simulink model "actuator_control_with_torque_commands"  (R2015a)
settings: Solver=FixedStepDiscrete  StartTime=0.0  StopTime=inf  FixedStep=sample_time  RelTol=1e-3
undefined symbols (not defined in the file): A1_notch_f1, A2_notch_f1, B1_notch_f1, B2_notch_f1, fdesignblkfcn, gcbh, K_notch_f1, k_sea_low, lateral_motor_efficiency, max_sagittal_unloaded_torque, sample_time
libraries: slrtlib x4
settings Model: CovSFcnEnable=off  Creator=wmartin  LastModifiedBy=wmartin
settings SolverCC: EnableConcurrentExecution=on
settings DataIOCC: MaxDataPoints=1000000000  SaveFormat=StructureWithTime  SaveOutput=off  SaveTime=off
settings OptimizationCC: BlockReduction=off  OptimizeBlockIOStorage=off  BufferReuse=off  GlobalBufferReuse=off  ExpressionFolding=off  LocalBlockOutputs=off  SimCompilerOptimization=on
settings DebuggingCC: SolverPrmCheckMsg=warning
settings HardwareCC: ProdIntDivRoundTo=Zero  ProdEndianess=LittleEndian  ProdLongLongMode=on  ProdHWDeviceType=Generic->32-bit x86 compatible
settings ModelReferenceCC: UpdateModelReferenceTargets=AssumeUpToDate  ModelReferenceNumInstancesAllowed=Single  ModelReferenceMinAlgLoopOccurrences=on
settings RTWCC: SystemTargetFile=slrt.tlc  TemplateMakefile=slrt_default_tmf  Description=Simulink Real-Time  RTWVerbose=off  RTWCompilerOptimization=on
settings SimulinkRealTimeCC: GeneratePreprocessorConditionals=Disable all

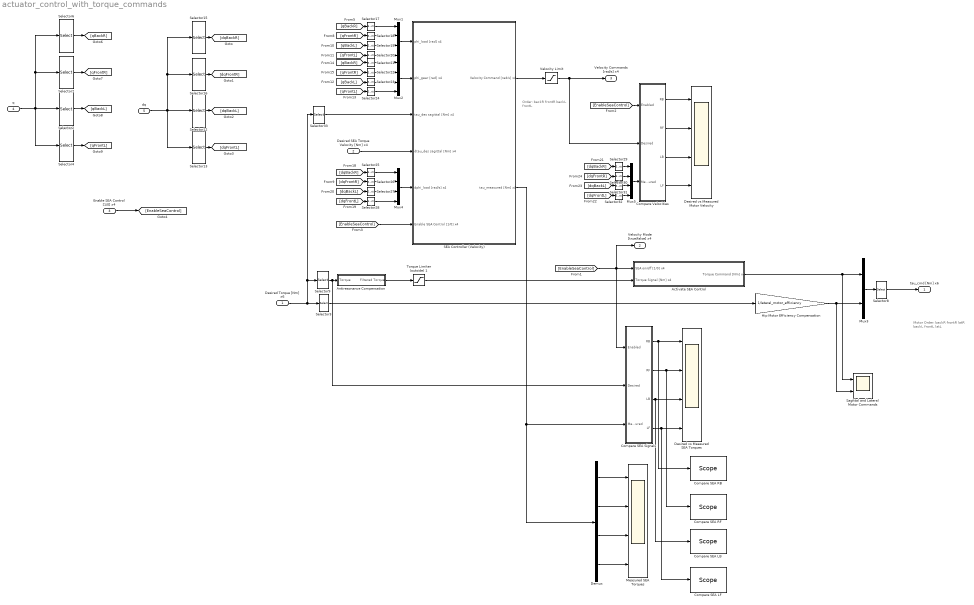
== system actuator_control_with_torque_commands ==
  note: Order:
      | backR
      | frontR
      | backL
      | frontL
  note: Motor Order:
      |
      | backR
      | frontR
      | latR
      | backL
      | frontL
      | latL
  Desired Torque [Nm] x6 : Inport  OutDataTypeStr=double  PortDimensions=6  SampleTime=sample_time
  Desired SEA Torque Velocity [Nm] x4 : Inport  Port=2  OutDataTypeStr=double  PortDimensions=4  SampleTime=sample_time
  Enable SEA Control [1/0] x4 : Inport  Port=3  OutDataTypeStr=boolean  PortDimensions=4  SampleTime=sample_time
  q : Inport  Port=4  OutDataTypeStr=double  PortDimensions=13  SampleTime=sample_time
  dq : Inport  Port=5  OutDataTypeStr=double  PortDimensions=13  SampleTime=sample_time
  Activate SEA Control : Subsystem
  Antiresonance Compensation : Subsystem
  Compare SEA LB : slrtlib/Displays and Logging/Scope   scopeno=3  scopetype=Host  autostart=on  viewmode=Graphical redraw  formatstr='%15.6f'  grid=on  ylimits=[0,0]  nosamples=1000  noprepostsamples=0  interleave=4  triggermode=FreeRun  triggersignal=1  trigsignalfromport=off  triggerlevel=0.0  triggerslope=Either  triggerscope=1  triggersample=0  filename=data.dat  mode=Lazy  writesize=512  autorestart=off  dynamicfilemode=off  maxwritefilesize=512*1024^2
  Compare SEA LF : slrtlib/Displays and Logging/Scope   scopeno=4  scopetype=Host  autostart=on  viewmode=Graphical redraw  formatstr='%15.6f'  grid=on  ylimits=[0,0]  nosamples=1000  noprepostsamples=0  interleave=4  triggermode=FreeRun  triggersignal=1  trigsignalfromport=off  triggerlevel=0.0  triggerslope=Either  triggerscope=1  triggersample=0  filename=data.dat  mode=Lazy  writesize=512  autorestart=off  dynamicfilemode=off  maxwritefilesize=512*1024^2
  "Compare SEA RB " : slrtlib/Displays and Logging/Scope   scopeno=1  scopetype=Host  autostart=on  viewmode=Graphical redraw  formatstr='%15.6f'  grid=on  ylimits=[0,0]  nosamples=1000  noprepostsamples=0  interleave=4  triggermode=FreeRun  triggersignal=1  trigsignalfromport=off  triggerlevel=0.0  triggerslope=Either  triggerscope=1  triggersample=0  filename=data.dat  mode=Lazy  writesize=512  autorestart=off  dynamicfilemode=off  maxwritefilesize=512*1024^2
  Compare SEA RF : slrtlib/Displays and Logging/Scope   scopeno=2  scopetype=Host  autostart=on  viewmode=Graphical redraw  formatstr='%15.6f'  grid=on  ylimits=[0,0]  nosamples=1000  noprepostsamples=0  interleave=4  triggermode=FreeRun  triggersignal=1  trigsignalfromport=off  triggerlevel=0.0  triggerslope=Either  triggerscope=1  triggersample=0  filename=data.dat  mode=Lazy  writesize=512  autorestart=off  dynamicfilemode=off  maxwritefilesize=512*1024^2
  Compare SEA Signals : Subsystem
  Compare Velocities : Subsystem
  Demux : Demux
  Desired vs Measured Motor Velocity : Scope  NumInputPorts=4
      settings: YMin=-0.3~-1~-1~-1  YMax=0.9~1~1~1  SaveName=ScopeData14  SampleInput=on
  Desired vs Measured SEA Torques : Scope  NumInputPorts=4
      settings: YMin=-1~-1~-200~70  YMax=1~1~-80~230  SaveName=SeaTorques  SampleInput=on  SampleTime=sample_time
  Hip Motor Efficiency Compensation : Gain  Gain=1/lateral_motor_efficiency
  Measured SEA Torques : Scope  NumInputPorts=4
      settings: YMin=-200~-350~-300~-150  YMax=50~50~50~200  SampleInput=on
  Mux{1..2,4..5} (4 alike) : Mux
  Mux3 : Mux  Inputs=2
  SEA Controller (Velocity) : Subsystem
  Sagittal and Lateral Motor Commands : Scope  NumInputPorts=2
      settings: YMin=-800~5  YMax=700~110  SaveName=ScopeData2  SampleInput=on
  Selector12 : Selector  InputPortWidth=13  Indices=[5 6]
  Selector13 : Selector  InputPortWidth=13  Indices=[7 8]
  Selector15 : Selector  InputPortWidth=13  Indices=[1 2]
  Selector16 : Selector  InputPortWidth=13  Indices=[3 4]
  Selector{17..20,25..28} (8 alike) : Selector  InputPortWidth=2  Indices=[1]
  Selector2 : Selector  InputPortWidth=13  Indices=[5 6]
  Selector{21..24,29..32} (8 alike) : Selector  InputPortWidth=2  Indices=[2]
  Selector3 : Selector  InputPortWidth=6  Indices=[3 6]
  Selector33 : Selector  InputPortWidth=6  Indices=[1 2 4 5]
  Selector4 : Selector  InputPortWidth=13  Indices=[7 8]
  Selector6 : Selector  InputPortWidth=13  Indices=[1 2]
  Selector7 : Selector  InputPortWidth=13  Indices=[3 4]
  Selector8 : Selector  InputPortWidth=6  Indices=[1 2 5 3 4 6]
  Selector9 : Selector  InputPortWidth=6  Indices=[1 2 4 5]
  Torque Limiter (outside) 1 : Saturate  UpperLimit=max_sagittal_unloaded_torque  LowerLimit=-max_sagittal_unloaded_torque
      settings: AttributesFormatString=Hi: %<UpperLimit>\nLo: %<LowerLimit>
  Velocity Limit : Saturate  UpperLimit=3  LowerLimit=-3
      settings: AttributesFormatString=Hi: %<UpperLimit>\nLo: %<LowerLimit>
  tau_cmd [Nm] x6 : Outport  OutDataTypeStr=double  PortDimensions=6  SampleTime=0  InitialOutput=[0 0 0 0 0 0]
  Velocity Mode [true/false] x4 : Outport  Port=2  InitialOutput=[false false false false]
  Velocity Commands [rad/s] x4 : Outport  Port=3  InitialOutput=[0 0 0 0]
  wires:
  Selector9/1 -> Compare SEA Signals/2(Desired), Antiresonance Compensation/1(Torque)
  SEA Controller (Velocity)/2(tau_measured [Nm] x4) -> Demux/1, Compare SEA Signals/3(Measured)
  Torque Limiter (outside) 1/1 -> Activate SEA Control/2(Torque Signal [Nm] x4)
  Desired Torque [Nm] x6/1 -> Selector33/1, Selector9/1, Selector3/1
  Selector8/1 -> tau_cmd [Nm] x6/1
  Selector6/1 -> [qBackR]
  Selector7/1 -> [qFrontR]
  Selector2/1 -> [qBackL]
  Selector4/1 -> [qFrontL]
  q/1 -> Selector2/1, Selector7/1, Selector6/1, Selector4/1
  dq/1 -> Selector13/1, Selector15/1, Selector16/1, Selector12/1
  Selector15/1 -> [dqBackR]
  Selector16/1 -> [dqFrontR]
  Selector12/1 -> [dqBackL]
  Selector13/1 -> [dqFrontL]
  Mux1/1 -> SEA Controller (Velocity)/1(phi_load [rad] x4)
  [qBackR] -> Selector17/1
  Selector17/1 -> Mux1/1
  Selector19/1 -> Mux1/3
  Selector18/1 -> Mux1/2
  Selector20/1 -> Mux1/4
  [qFrontR] -> Selector18/1
  [qBackL] -> Selector19/1
  [qFrontL] -> Selector20/1
  Mux2/1 -> SEA Controller (Velocity)/2(phi_gear [rad] x4)
  [qBackR] -> Selector21/1
  Selector21/1 -> Mux2/1
  Selector23/1 -> Mux2/3
  Selector22/1 -> Mux2/2
  Selector24/1 -> Mux2/4
  [qFrontR] -> Selector22/1
  [qBackL] -> Selector23/1
  [qFrontL] -> Selector24/1
  Mux4/1 -> SEA Controller (Velocity)/5(dphi_load [rad/s] x4)
  [dqBackR] -> Selector25/1
  Selector25/1 -> Mux4/1
  Selector27/1 -> Mux4/3
  Selector26/1 -> Mux4/2
  Selector28/1 -> Mux4/4
  [dqFrontR] -> Selector26/1
  [dqBackL] -> Selector27/1
  [dqFrontL] -> Selector28/1
  Mux5/1 -> Compare Velocities/3(Measured)
  [dqBackR] -> Selector29/1
  Selector29/1 -> Mux5/1
  Selector31/1 -> Mux5/3
  Selector30/1 -> Mux5/2
  Selector32/1 -> Mux5/4
  [dqFrontR] -> Selector30/1
  [dqBackL] -> Selector31/1
  [dqFrontL] -> Selector32/1
  Selector33/1 -> SEA Controller (Velocity)/3(tau_des sagittal [Nm] x4)
  Selector3/1 -> Hip Motor Efficiency Compensation/1
  Mux3/1 -> Selector8/1
  Antiresonance Compensation/1(Filtered Torque) -> Torque Limiter (outside) 1/1
  Desired SEA Torque Velocity [Nm] x4/1 -> SEA Controller (Velocity)/4(dtau_des sagittal [Nm] x4)
  Activate SEA Control/1(Torque Command [Nm] x4) -> Sagittal and Lateral Motor Commands/1, Mux3/1
  Hip Motor Efficiency Compensation/1 -> Sagittal and Lateral Motor Commands/2, Mux3/2
  Compare SEA Signals/1(RB) -> "Compare SEA RB "/1, Desired vs Measured SEA Torques/1
  Compare SEA Signals/2(RF) -> Desired vs Measured SEA Torques/2, Compare SEA RF/1
  Demux/1 -> Measured SEA Torques/1
  Demux/2 -> Measured SEA Torques/2
  Demux/3 -> Measured SEA Torques/3
  Demux/4 -> Measured SEA Torques/4
  Compare SEA Signals/3(LB) -> Compare SEA LB/1, Desired vs Measured SEA Torques/3
  Compare SEA Signals/4(LF) -> Desired vs Measured SEA Torques/4, Compare SEA LF/1
  SEA Controller (Velocity)/1(Velocity Command [rad/s] x4) -> Velocity Limit/1
  [EnableSeaControl] -> Compare SEA Signals/1(Enabled), Velocity Mode [true/false] x4/1, Activate SEA Control/1("SEA on/off [1/0] x4 ")
  Compare Velocities/4(LF) -> Desired vs Measured Motor Velocity/4
  Compare Velocities/3(LB) -> Desired vs Measured Motor Velocity/3
  Compare Velocities/1(RB) -> Desired vs Measured Motor Velocity/1
  Compare Velocities/2(RF) -> Desired vs Measured Motor Velocity/2
  Enable SEA Control [1/0] x4/1 -> [EnableSeaControl]
  [EnableSeaControl] -> Compare Velocities/1(Enabled)
  [EnableSeaControl] -> SEA Controller (Velocity)/6(Enable SEA Control [1/0] x4)
  Velocity Limit/1 -> Compare Velocities/2(Desired), Velocity Commands [rad/s] x4/1

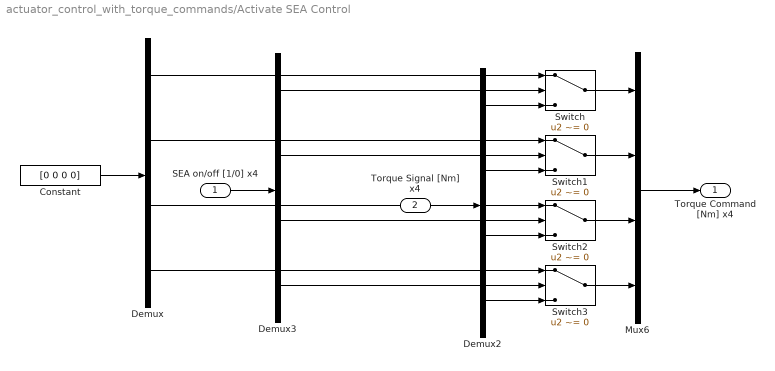
== system actuator_control_with_torque_commands/Activate SEA Control ==
  "SEA on/off [1/0] x4 " : Inport
  Torque Signal [Nm] x4 : Inport  Port=2
  Constant : Constant  Value=[0 0 0 0]
  Demux : Demux
  Demux2 : Demux
  Demux3 : Demux
  Mux6 : Mux
  Switch{,1..3} (4 alike) : Switch  Criteria=u2 ~= 0
  Torque Command [Nm] x4 : Outport
  wires:
  Demux2/2 -> Switch1/3
  Demux2/1 -> Switch/3
  Demux/1 -> Switch/1
  Switch/1 -> Mux6/1
  Switch1/1 -> Mux6/2
  Switch3/1 -> Mux6/4
  Demux3/1 -> Switch/2
  Mux6/1 -> Torque Command [Nm] x4/1
  Demux3/3 -> Switch2/2
  Demux3/2 -> Switch1/2
  Demux/3 -> Switch2/1
  Switch2/1 -> Mux6/3
  Demux/4 -> Switch3/1
  Demux2/4 -> Switch3/3
  Demux3/4 -> Switch3/2
  Demux/2 -> Switch1/1
  Demux2/3 -> Switch2/3
  Constant/1 -> Demux/1
  "SEA on/off [1/0] x4 "/1 -> Demux3/1
  Torque Signal [Nm] x4/1 -> Demux2/1

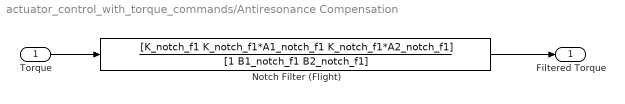
== system actuator_control_with_torque_commands/Antiresonance Compensation ==
  Torque : Inport
  Notch Filter (Flight) : DiscreteTransferFcn  Numerator=[K_notch_f1 K_notch_f1*A1_notch_f1 K_notch_f1*A2_notch_f1]  Denominator=[1 B1_notch_f1 B2_notch_f1]  SampleTime=sample_time
  Filtered Torque : Outport
  wires:
  Torque/1 -> Notch Filter (Flight)/1
  Notch Filter (Flight)/1 -> Filtered Torque/1

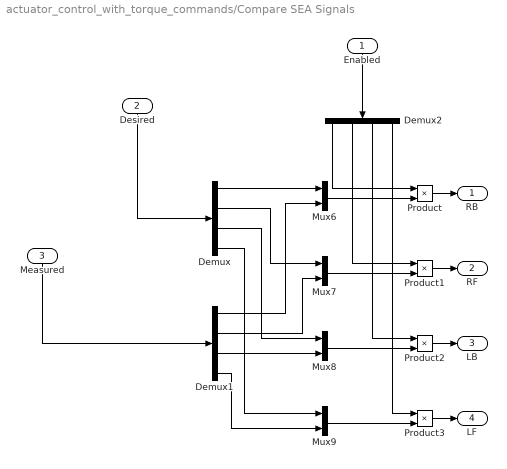
== system actuator_control_with_torque_commands/Compare SEA Signals ==
  Enabled : Inport
  Desired : Inport  Port=2
  Measured : Inport  Port=3
  Demux : Demux
  Demux1 : Demux
  Demux2 : Demux
  Mux{6..9} (4 alike) : Mux  Inputs=2
  Product{,1..3} (4 alike) : Product
  RB : Outport
  RF : Outport  Port=2
  LB : Outport  Port=3
  LF : Outport  Port=4
  wires:
  Demux/3 -> Mux8/1
  Demux/2 -> Mux7/1
  Demux1/1 -> Mux6/2
  Demux/1 -> Mux6/1
  Product/1 -> RB/1
  Demux/4 -> Mux9/1
  Mux6/1 -> Product/2
  Demux1/4 -> Mux9/2
  Mux7/1 -> Product1/2
  Mux9/1 -> Product3/2
  Measured/1 -> Demux1/1
  Demux2/3 -> Product2/1
  Demux1/2 -> Mux7/2
  Desired/1 -> Demux/1
  Demux2/1 -> Product/1
  Product3/1 -> LF/1
  Product1/1 -> RF/1
  Product2/1 -> LB/1
  Mux8/1 -> Product2/2
  Demux1/3 -> Mux8/2
  Enabled/1 -> Demux2/1
  Demux2/4 -> Product3/1
  Demux2/2 -> Product1/1

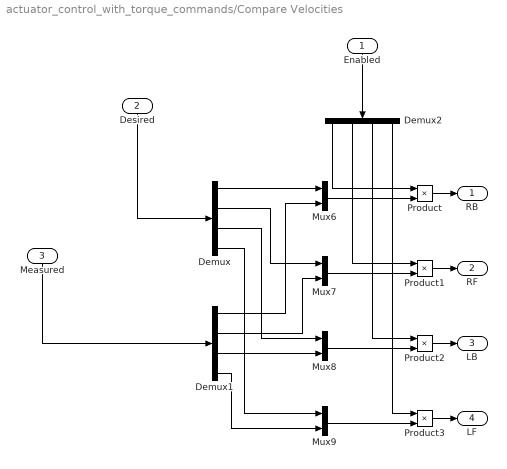
== system actuator_control_with_torque_commands/Compare Velocities ==
  Enabled : Inport
  Desired : Inport  Port=2
  Measured : Inport  Port=3
  Demux : Demux
  Demux1 : Demux
  Demux2 : Demux
  Mux{6..9} (4 alike) : Mux  Inputs=2
  Product{,1..3} (4 alike) : Product
  RB : Outport
  RF : Outport  Port=2
  LB : Outport  Port=3
  LF : Outport  Port=4
  wires:
  Demux2/2 -> Product1/1
  Demux2/4 -> Product3/1
  Enabled/1 -> Demux2/1
  Demux1/3 -> Mux8/2
  Mux8/1 -> Product2/2
  Product2/1 -> LB/1
  Product1/1 -> RF/1
  Product3/1 -> LF/1
  Demux2/1 -> Product/1
  Desired/1 -> Demux/1
  Demux1/2 -> Mux7/2
  Demux2/3 -> Product2/1
  Measured/1 -> Demux1/1
  Mux9/1 -> Product3/2
  Mux7/1 -> Product1/2
  Demux1/4 -> Mux9/2
  Mux6/1 -> Product/2
  Demux/4 -> Mux9/1
  Product/1 -> RB/1
  Demux/1 -> Mux6/1
  Demux1/1 -> Mux6/2
  Demux/2 -> Mux7/1
  Demux/3 -> Mux8/1

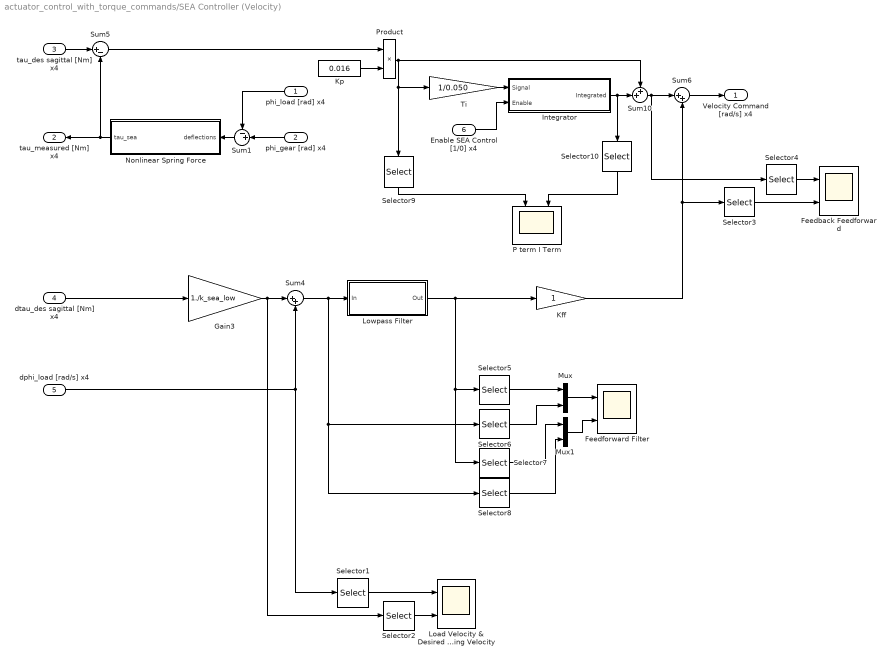
== system actuator_control_with_torque_commands/SEA Controller (Velocity) ==
  phi_load [rad] x4 : Inport
  phi_gear [rad] x4 : Inport  Port=2
  tau_des sagittal [Nm] x4 : Inport  Port=3
  dtau_des sagittal [Nm] x4 : Inport  Port=4
  dphi_load [rad/s] x4 : Inport  Port=5
  Enable SEA Control [1/0] x4 : Inport  Port=6
  Feedback Feedforward : Scope  NumInputPorts=2
      settings: YMin=-4~-0.9  YMax=4.5~1  SaveName=ScopeData7  SampleInput=on
  Feedforward Filter : Scope  NumInputPorts=2
      settings: YMin=-0.15~-0.2  YMax=0.1~0.45  SaveName=ScopeData3  SampleInput=on
  Gain3 : Gain  Gain=1./k_sea_low
  Integrator : Subsystem
  Kff : Gain
  Kp : Constant  Value=0.016
  Load Velocity & Desired Spring Velocity : Scope  NumInputPorts=2
      settings: YMin=-0.8~-0.15  YMax=0.8~0.15  SampleInput=on
  Lowpass Filter : Subsystem  DialogController=fdesignblkfcn  InitFcn=fdesignblkfcn(gcbh, {'InitFcn'});  mask(Lowpass Filter){}
      mask help: Design a lowpass filter
      settings: CopyFcn=fdesignblkfcn(gcbh, {'CopyFcn'});
      mask Help: helpview(mapfilelocation('dsp'), 'dsplowpassfilter');
      mask Display: disp('Lowpass')
  Mux : Mux  Inputs=2
  Mux1 : Mux  Inputs=2
  Nonlinear Spring Force : MATLAB Function  TreatAsAtomicUnit=on
  P term I Term : Scope  NumInputPorts=2
      settings: YMin=-0.4~-0.15  YMax=1.7~1  SaveName=ScopeData4  SampleInput=on
  Product : Product
  Selector{1..4,9..10} (6 alike) : Selector  InputPortWidth=4  Indices=[1 2]
  Selector5 : Selector  InputPortWidth=4  Indices=[1]
  Selector6 : Selector  InputPortWidth=4  Indices=[1]
  Selector7 : Selector  InputPortWidth=4  Indices=[2]
  Selector8 : Selector  InputPortWidth=4  Indices=[2]
  Sum1 : Sum  Inputs=-+|
  Sum10 : Sum  Inputs=++|
  Sum4 : Sum  Inputs=|++
  Sum5 : Sum  Inputs=|+-
  Sum6 : Sum  Inputs=|++
  Ti : Gain  Gain=1/0.050
  Velocity Command [rad/s] x4 : Outport
  tau_measured [Nm] x4 : Outport  Port=2
  wires:
  Sum1/1 -> Nonlinear Spring Force/1(deflections)
  Nonlinear Spring Force/1(tau_sea) -> Sum5/2, tau_measured [Nm] x4/1
  phi_load [rad] x4/1 -> Sum1/1
  phi_gear [rad] x4/1 -> Sum1/2
  tau_des sagittal [Nm] x4/1 -> Sum5/1
  Sum10/1 -> Selector4/1, Sum6/1
  Product/1 -> Ti/1, Selector9/1, Sum10/1
  Sum6/1 -> Velocity Command [rad/s] x4/1
  Kp/1 -> Product/2
  Selector3/1 -> Feedback Feedforward/2
  Gain3/1 -> Sum4/1, Selector2/1
  dtau_des sagittal [Nm] x4/1 -> Gain3/1
  Enable SEA Control [1/0] x4/1 -> Integrator/2(Enable)
  Sum5/1 -> Product/1
  Integrator/1(Integrated) -> Sum10/2, Selector10/1
  Ti/1 -> Integrator/1(Signal)
  Selector1/1 -> Load Velocity & Desired Spring Velocity/1
  Selector2/1 -> Load Velocity & Desired Spring Velocity/2
  Selector4/1 -> Feedback Feedforward/1
  dphi_load [rad/s] x4/1 -> Sum4/2, Selector1/1
  Selector5/1 -> Mux/1
  Selector6/1 -> Mux/2
  Mux/1 -> Feedforward Filter/1
  Mux1/1 -> Feedforward Filter/2
  Selector7/1 -> Mux1/1
  Selector8/1 -> Mux1/2
  Sum4/1 -> Selector8/1, Selector6/1, Lowpass Filter/1(In)
  Lowpass Filter/1(Out) -> Selector5/1, Selector7/1, Kff/1
  Kff/1 -> Selector3/1, Sum6/2
  Selector9/1 -> P term I Term/1
  Selector10/1 -> P term I Term/2

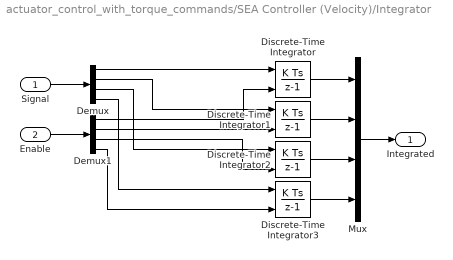
== system actuator_control_with_torque_commands/SEA Controller (Velocity)/Integrator ==
  Signal : Inport
  Enable : Inport  Port=2
  Demux : Demux
  Demux1 : Demux
  Discrete-Time Integrator{,1..3} (4 alike) : DiscreteIntegrator  ExternalReset=rising  InitialConditionSetting=State (most efficient)  SampleTime=sample_time  LimitOutput=on  UpperSaturationLimit=1  LowerSaturationLimit=-1
  Mux : Mux
  Integrated : Outport
  wires:
  Signal/1 -> Demux/1
  Discrete-Time Integrator/1 -> Mux/1
  Enable/1 -> Demux1/1
  Mux/1 -> Integrated/1
  Discrete-Time Integrator1/1 -> Mux/2
  Discrete-Time Integrator2/1 -> Mux/3
  Discrete-Time Integrator3/1 -> Mux/4
  Demux1/4 -> Discrete-Time Integrator3/2
  Demux1/3 -> Discrete-Time Integrator2/2
  Demux1/2 -> Discrete-Time Integrator1/2
  Demux1/1 -> Discrete-Time Integrator/2
  Demux/1 -> Discrete-Time Integrator/1
  Demux/2 -> Discrete-Time Integrator1/1
  Demux/3 -> Discrete-Time Integrator2/1
  Demux/4 -> Discrete-Time Integrator3/1

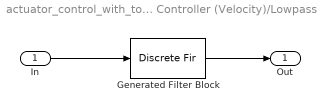
== system actuator_control_with_torque_commands/SEA Controller (Velocity)/Lowpass Filter ==
  In : Inport
  Generated Filter Block : DiscreteFir  Tag=BlockMethodSubSystem  Coefficients=[-0.049792265798371309 -0.00478204397482343 -0.0023545966524627579 0.0019617877955006649 0.0081617445920188422 0.01606136498204886 0.025426522925330174 0.035808512742994333 0.046780148761454213 0.057713212050140641 0.068077289761393753 0.077169075575072327 0.084565882051693325 0.089692876147162801 0.092473878579640248 0.092473878579640248 0.089692876147162801 0.084565882051693325 0.077169075575072327 0.068077289761393753 0.057713212050140641 0.046780148761454213 0.035808512742994333 0.025426522925330174 0.01606136498204886 0.0081617445920188422 0.0019617877955006649 -0.0023545966524627579 -0.00478204397482343 -0.049792265798371309]
  Out : Outport
  wires:
  In/1 -> Generated Filter Block/1
  Generated Filter Block/1 -> Out/1

== matlab function actuator_control_with_torque_commands/SEA Controller (Velocity)/Nonlinear Spring Force ==
  data: deflections input; tau_sea output
function tau_sea   = SeaSpringForce( deflections )
    tau_sea = SeaSpringForce( deflections );
end
